simulink model "SkywaveAutopilot"  (R2024b)
settings: Solver=ode45  StartTime=0.0  StopTime=2500  FixedStep=.01  MaxStep=.004  RelTol=1e-5  EnableMultiTasking=on
values from neighbouring files (symbols this model uses):
  ac = [xcg - 0.25 * cbar, 0, 0]    [SkyWaveGeom.m]
  b = 70    [SkyWaveGeom.m]
  cbar = 10    [SkyWaveGeom.m]
  cda2 = 0.33    [SkyWaveGeom.m]
  cdo = 0.05    [SkyWaveGeom.m]
  cg = [xcg 0 0]    [SkyWaveGeom.m]
  cla = 4.44    [SkyWaveGeom.m]
  cladot = 0    [SkyWaveGeom.m]
  clb = -0.074    [SkyWaveGeom.m]
  clda = -0.134    [SkyWaveGeom.m]
  clde = 0.355    [SkyWaveGeom.m]
  cldr = 0.107    [SkyWaveGeom.m]
  clo = 0.41    [SkyWaveGeom.m]
  clp = -0.410    (= -0.41)    [SkyWaveGeom.m]
  clq = 3.8    [SkyWaveGeom.m]
  clr = 0.107    [SkyWaveGeom.m]
  cma = -0.683    [SkyWaveGeom.m]
  cmadot = -4.36    [SkyWaveGeom.m]
  cmde = -0.923    [SkyWaveGeom.m]
  cmq = -9.96    [SkyWaveGeom.m]
  cnb = 0.071    [SkyWaveGeom.m]
  cnda = -0.0035    [SkyWaveGeom.m]
  cndr = -0.072    [SkyWaveGeom.m]
  cnp = -0.0575    [SkyWaveGeom.m]
  cnr = -0.125    [SkyWaveGeom.m]
  cyb = -0.564    [SkyWaveGeom.m]
  cydr = 0.157    [SkyWaveGeom.m]
  eng = [xcg 0 0]    [SkyWaveGeom.m]
  initalt = 5000    [SkyWaveGeom.m]
  initbank = 0    [SkyWaveGeom.m]
  initeast = 0    [SkyWaveGeom.m]
  inithead = 0 * pi / 180    (= 0)    [SkyWaveGeom.m]
  initnorth = 0    [SkyWaveGeom.m]
  initp = 0    [SkyWaveGeom.m]
  initpitch = initw / initu    (= -0.0272251308901)    [SkyWaveGeom.m]
  initq = 0    [SkyWaveGeom.m]
  initr = 0    [SkyWaveGeom.m]
  initu = 238.75    [SkyWaveGeom.m]
  initv = 0    [SkyWaveGeom.m]
  initw = -6.5    [SkyWaveGeom.m]
  jx = 0.25 * mass * (b/2)^2    (= 247282.608696)    [SkyWaveGeom.m]
  jxz = 0    [SkyWaveGeom.m]
  jy = 0.35 * mass * (cbar)^2    (= 28260.8695652)    [SkyWaveGeom.m]
  jz = 0.5 * mass * (b/2)^2    (= 494565.217391)    [SkyWaveGeom.m]
  sw = 700    [SkyWaveGeom.m]
  weight = 26000    [SkyWaveGeom.m]
libraries: slpidlib x7, simulink_extras x5, aerolibfltsims x2, dspswit3 x1, vrlib x1, aerolibanimutils x1
(part 1 of 2)
settings Model: SimulationMode=accelerator  Creator=andersop  LastModifiedBy=gigi
settings SolverCC: InitialStep=.004  AlgebraicLoopSolver=TrustRegion
settings DataIOCC: LimitDataPoints=on  SaveFormat=Array  SignalLoggingSaveFormat=ModelDataLogs  SaveState=on  ReturnWorkspaceOutputs=off  SignalLoggingName=sigsOut
settings OptimizationCC: ExpressionDepthLimit=2147483647  InitFltsAndDblsToZero=on  LifeSpan=inf
settings DebuggingCC: SaveWithParameterizedLinksMsg=none  UnderspecifiedInitializationDetection=Classic  MergeDetectMultiDrivingBlocksExec=none  SignalResolutionControl=TryResolveAllWithWarning  MultiTaskDSMMsg=warning  MultiTaskCondExecSysMsg=none  FcnCallInpInsideContextMsg=warning  UnconnectedInputMsg=warning  UnconnectedOutputMsg=warning  UnconnectedLineMsg=warning  StateNameClashWarn=warning  SFUnexpectedBacktrackingDiag=warning  SFNoUnconditionalDefaultTransitionDiag=warning  SFExecutionAtInitializationDiag=none  ArithmeticOperatorsInVariantConditions=warning
settings HardwareCC: ProdBitPerPointer=32  ProdBitPerSizeT=32  ProdBitPerPtrDiffT=32  ProdLargestAtomicFloat=None  ProdIntDivRoundTo=Undefined  ProdEndianess=Unspecified  ProdWordSize=32  ProdHWDeviceType=32-bit Generic  TargetUnknown=on
settings ModelReferenceCC: PropagateSignalLabelsOutOfModel=off
settings SFSimCC: SimUseLocalCustomCode=off  CustomCodeUndefinedFunction=UseInterfaceOnly
settings RTWCC: RTWUseLocalCustomCode=off  GPUComputeCapability=3.5
settings CodeAppCC: StateflowObjectComments=on
settings GRTTargetCC: TargetFcnLib=ansi_tfl_tmw.mat  TargetLangStandard=C89/C90 (ANSI)  ModelReferenceCompliant=off  CombineOutputUpdateFcns=off  MatFileLogging=off  GRTInterface=on
settings ConfigComp: CovMetricSettings=dw  CovSaveCumulativeToWorkspaceVar=on  CovSaveSingleToWorkspaceVar=on  CovExternalEMLEnable=off

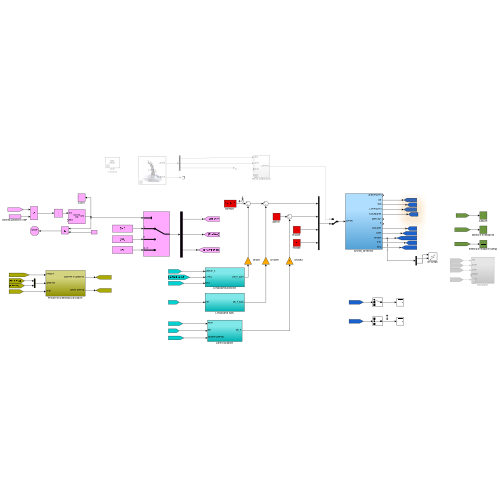
[thumbnail: Simulink's stored preview of the top-level diagram]
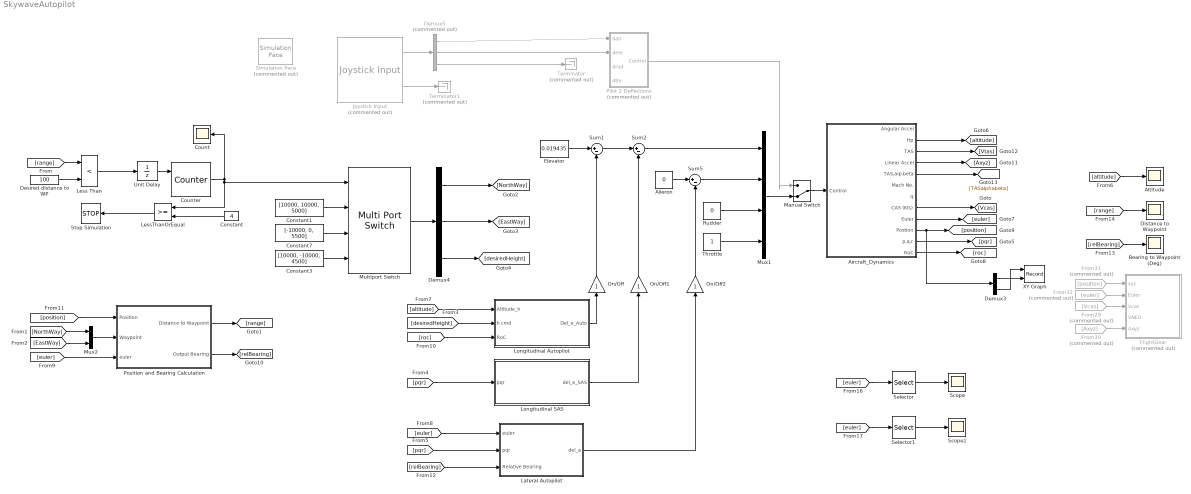
== system SkywaveAutopilot ==
  Aileron : Constant  Value=0
  Aircraft_Dynamics : Subsystem
  Altitude : Scope
  Bearing to Waypoint (Deg) : Scope
  Constant : Constant  Value=4
  Constant1 : Constant  Value=[10000, 10000, 5000]
  Constant3 : Constant  Value=[10000, -10000, 4500]
  Constant7 : Constant  Value=[-10000, 0, 5500]
  Count : Scope
  Counter : dspswit3/Counter  Direction=Up  CountEvent=Rising edge  CounterSize=User defined  MaxCount=255  InitialCount=1  Output=Count  HitValue=32  ResetInput=on  SamplesPerFrame=1  Ts=1  CntDtype=double  HitDtype=Logical
  Demux3 : Demux  Outputs=2
  Demux4 : Demux  Outputs=3
  Demux5 : Demux  Commented=on  Outputs=[1 1 2]
  Desired distance to WP : Constant  Value=100
  Distance to Waypoint : Scope
  Elevator : Constant  Value=0.019435
  FlightGear : Subsystem  Commented=on
  From29 : From  Commented=on  GotoTag=Vcas
  From30 : From  Commented=on  GotoTag=Axyz
  From31 : From  Commented=on  GotoTag=position
  From32 : From  Commented=on  GotoTag=euler
  Joystick Input : vrlib/Joystick Input  Commented=on  joyid=2  adjustports=on  forcefeed=off
  Lateral Autopilot : Subsystem
  Less Than : RelationalOperator  Operator=<  OutDataTypeStr=boolean  RndMeth=Simplest  InputSameDT=off
  LessThanOrEqual : RelationalOperator  OutDataTypeStr=boolean  RndMeth=Simplest  InputSameDT=off
  Longitudinal Autopilot : Subsystem
  Longitudinal SAS : Subsystem
  Manual Switch : ManualSwitch  CurrentSetting=0
  Multiport Switch : MultiPortSwitch  DiagnosticForDefault=None  SaturateOnIntegerOverflow=off  InputSameDT=off
  Mux1 : Mux
  Mux2 : Mux  Inputs=2
  On/Off : Gain
  On/Off1 : Gain
  On/Off2 : Gain
  Pilot 2 Deflections : Subsystem  Commented=on
  Position and Bearing Calculation : Subsystem
  Rudder : Constant  Value=0
  Scope : Scope
  Scope1 : Scope
  Selector : Selector  InputPortWidth=3  IndexOptions=Index vector (dialog)  Indices=[1]  OutputSizes=1
  Selector1 : Selector  InputPortWidth=3  IndexOptions=Index vector (dialog)  Indices=[2]  OutputSizes=1
  Simulation Pace : aerolibanimutils/Simulation Pace  Commented=on  SimulationPace=1  SleepMode=Auto  OutputPaceError=off  SampleTime=1/30
  Stop Simulation : Stop
  Sum1 : Sum  Inputs=|+-
  Sum2 : Sum  Inputs=|+-
  Sum5 : Sum  Inputs=|+-
  Terminator : Terminator  Commented=on
  Terminator1 : Terminator  Commented=on
  Throttle : Constant
  Unit Delay : UnitDelay  InitialCondition=1  SampleTime=-1  HasFrameUpgradeWarning=on
  XY Graph : Record  FileSettingsInternal="{\"entries\":[{\"content\":{\"excelSettings\":{\"content\":{},\"type\":\"Streamout.ExcelSettings\"}},\"type\":\"Streamout.FileSettingStorage\",\"uuid\":\"\"}],\"packageUris\":[\"http:\\/\\/schema.mathworks.com\\/mf0\\/streamout_blocks\\/R2020a\"],\"version\":\"1.0\"}"  Layout=[1 1]  SignalsInternal="{\"entries\":[{\"content\":{\"signals\":[{\"content\":{\"blockPath\":[],\"dimensions\":[1],\"domain\":\"\",\"lineColor\":\"#a2142f\",\"port\":1,\"sid\":[\"\"],\"signalID\":1,\"signalName\":\"Demux3:2\"},\"type\":\"RecordBlkView.Signal\",\"uuid\":\"\"},{\"content\":{\"blockPath\":[],\"dimensions\":[2],\"domain\":\"\",\"hasChildren\":true,\"lineColor\":\"#d95319\",\"lineWidth\":2,\"port\":2,\"sid\":[\"\"],\"signalID\":2,\"signalName\":\"Demux3:1\"},\"type\":\"RecordBlkView.Signal\",\"uuid\":\"\"},{\"content\":{\"blockPath\":[],\"channel\":[1],\"dimensions\":[2],\"domain\":\"\",\"lineColor\":\"#a2142f\",\"lineWidth\":2,\"parentID\":2,\"plots\":[ 1 ],\"port\":2,\"sid\":[\"\"],\"signalID\":3,\"signalName\":\"Demux3:1\"},\"type\":\"RecordBlkView.Signal\",\"uuid\":\"\"},{\"content\":{\"blockPath\":[],\"channel\":[2],\"dimensions\":[2],\"domain\":\"\",\"lineColor\":\"#139fff\",\"lineWidth\":2,\"parentID\":2,\"plots\":[ 1 ],\"port\":2,\"sid\":[\"\"],\"signalID\":4,\"signalName\":\"Demux3:1\"},\"type\":\"RecordBlkView.Signal\",\"uuid\":\"\"}]},\"type\":\"RecordBlkView.InputSignals\",\"uuid\":\"\"}],\"packageUris\":[\"http:\\/\\/schema.mathworks.com\\/mf0\\/streamout_blocks\\/R2020a\"],\"version\":\"1.0\"}"  VisualizationBindings="{\"xyplotplugin\":{\"info\":[{\"series\":[{\"bindingParametersList\":[{\"parameter\":\"X-Axis\",\"signalID\":4,\"signalName\":\"Demux3:1(2)\"},{\"parameter\":\"Y-Axis\",\"signalID\":3,\"signalName\":\"Demux3:1(1)\"}],\"seriesID\":0}],\"subplotID\":1}]}}"  CompatibilityTag=XY
  wires:
  Aircraft_Dynamics/9(Euler) -> [euler]
  Elevator/1 -> Sum1/1
  On/Off/1 -> Sum1/2
  Sum1/1 -> Sum2/1
  On/Off1/1 -> Sum2/2
  Aircraft_Dynamics/10(Postion) -> Demux3/1, [position]
  Position and Bearing Calculation/1(Distance to Waypoint) -> [range]
  Position and Bearing Calculation/2(Output Bearing) -> [relBearing]
  Aileron/1 -> Sum5/1
  Sum5/1 -> Mux1/2
  On/Off2/1 -> Sum5/2
  Lateral Autopilot/1(del_a) -> On/Off2/1
  Counter/1 -> Multiport Switch/1, LessThanOrEqual/1, Count/1
  Less Than/1 -> Unit Delay/1
  Demux3/2 -> XY Graph/1
  Demux3/1 -> XY Graph/2
  Unit Delay/1 -> Counter/1
  Desired distance to WP/1 -> Less Than/2
  Constant/1 -> LessThanOrEqual/2
  LessThanOrEqual/1 -> Stop Simulation/1
  Constant1/1 -> Multiport Switch/2
  Constant7/1 -> Multiport Switch/3
  Constant3/1 -> Multiport Switch/4
  [range] -> Less Than/1
  Multiport Switch/1 -> Demux4/1
  Demux4/1 -> [NorthWay]
  Demux4/2 -> [EastWay]
  Demux4/3 -> [desiredHeight]
  Mux2/1 -> Position and Bearing Calculation/2(Waypoint)
  [NorthWay] -> Mux2/1
  [EastWay] -> Mux2/2
  [desiredHeight] -> Longitudinal Autopilot/2(h cmd)
  Aircraft_Dynamics/11(p,q,r) -> [pqr]
  [pqr] -> Longitudinal SAS/1(pqr)
  [pqr] -> Lateral Autopilot/2(pqr)
  Aircraft_Dynamics/2(Hp) -> [altitude]
  [altitude] -> Altitude/1
  [altitude] -> Longitudinal Autopilot/1(Altitude_h)
  [euler] -> Lateral Autopilot/1(euler)
  [euler] -> Position and Bearing Calculation/3(euler)
  Aircraft_Dynamics/12(RoC) -> [roc]
  [roc] -> Longitudinal Autopilot/3(RoC)
  [position] -> Position and Bearing Calculation/1(Position)
  [relBearing] -> Lateral Autopilot/3(Relative Bearing)
  [relBearing] -> Bearing to Waypoint (Deg)/1
  [range] -> Distance to Waypoint/1
  From32/1 -> FlightGear/2(Euler)
  From31/1 -> FlightGear/1(xyz)
  From29/1 -> FlightGear/3(Vcas)
  From30/1 -> FlightGear/5(Axyz)
  Demux5/2 -> Pilot 2 Deflections/2(dele)
  Joystick Input/2 -> Terminator1/1
  Demux5/3 -> Terminator/1
  Demux5/1 -> Pilot 2 Deflections/1(dail)
  Joystick Input/1 -> Demux5/1
  Mux1/1 -> Manual Switch/2
  Pilot 2 Deflections/1(Control) -> Manual Switch/1
  Manual Switch/1 -> Aircraft_Dynamics/1(Control)
  Aircraft_Dynamics/8(CAS (Kts)) -> [Vcas]
  Aircraft_Dynamics/4(Linear Accel) -> [Axyz]
  Aircraft_Dynamics/3(TAS) -> [Vtas]
  [euler] -> Selector/1
  Selector/1 -> Scope/1
  [euler] -> Selector1/1
  Selector1/1 -> Scope1/1
  Rudder/1 -> Mux1/3
  Sum2/1 -> Mux1/1
  Throttle/1 -> Mux1/4
  Longitudinal Autopilot/1(Del_e_Auto) -> On/Off/1
  Longitudinal SAS/1(del_e_SAS) -> On/Off1/1
  Aircraft_Dynamics/5(TAS,alp,beta) -> [TASalphabeta]

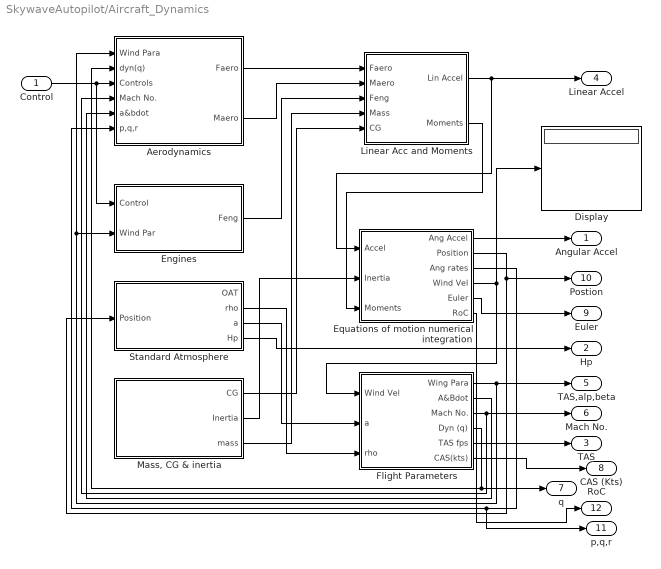
== system SkywaveAutopilot/Aircraft_Dynamics ==
  Control : Inport
  Aerodynamics : Subsystem
  Display : Display
  Engines : Subsystem
  "Equations of motion numerical integration " : Subsystem
  Flight Parameters : Subsystem
  Linear Acc and Moments : Subsystem
  "Mass, CG & inertia" : Subsystem
  Standard Atmosphere : Subsystem
  Angular Accel : Outport
  Hp : Outport  Port=2
  TAS : Outport  Port=3
  Linear Accel : Outport  Port=4
  TAS,alp,beta : Outport  Port=5
  Mach No. : Outport  Port=6
  q : Outport  Port=7
  CAS (Kts) : Outport  Port=8
  Euler : Outport  Port=9
  Postion : Outport  Port=10
  p,q,r : Outport  Port=11
  RoC : Outport  Port=12
  wires:
  Aerodynamics/1(Faero) -> Linear Acc and Moments/1(Faero)
  Aerodynamics/2(Maero) -> Linear Acc and Moments/2(Maero)
  Control/1 -> Aerodynamics/3(Controls), Engines/1(Control)
  Engines/1(Feng) -> Linear Acc and Moments/3(Feng)
  "Mass, CG & inertia"/1(CG) -> Linear Acc and Moments/5(CG)
  "Mass, CG & inertia"/2(Inertia) -> "Equations of motion numerical integration "/2(Inertia)
  Linear Acc and Moments/1(Lin Accel) -> "Equations of motion numerical integration "/1(Accel), Linear Accel/1
  Linear Acc and Moments/2(Moments) -> "Equations of motion numerical integration "/3(Moments)
  "Equations of motion numerical integration "/3(Ang rates) -> Aerodynamics/6(p,q,r), p,q,r/1
  "Equations of motion numerical integration "/4(Wind Vel) -> Display/1, Flight Parameters/1(Wind Vel)
  Flight Parameters/1(Wing Para) -> TAS,alp,beta/1, Aerodynamics/1(Wind Para), Engines/2(Wind Par)
  Flight Parameters/4(Dyn (q)) -> Aerodynamics/2(dyn(q)), q/1
  Flight Parameters/3(Mach No.) -> Mach No./1, Aerodynamics/4(Mach No.)
  Flight Parameters/2(A&Bdot) -> Aerodynamics/5(a&bdot)
  "Equations of motion numerical integration "/2(Position) -> Postion/1, Standard Atmosphere/1(Position)
  "Equations of motion numerical integration "/1(Ang Accel) -> Angular Accel/1
  Standard Atmosphere/4(Hp) -> Hp/1
  Flight Parameters/5(TAS fps) -> TAS/1
  Flight Parameters/6(CAS(kts)) -> CAS (Kts)/1
  "Equations of motion numerical integration "/5(Euler) -> Euler/1
  Standard Atmosphere/3(a) -> Flight Parameters/2(a)
  Standard Atmosphere/2(rho) -> Flight Parameters/3(rho)
  "Mass, CG & inertia"/3(mass) -> Linear Acc and Moments/4(Mass)
  "Equations of motion numerical integration "/6(RoC) -> RoC/1

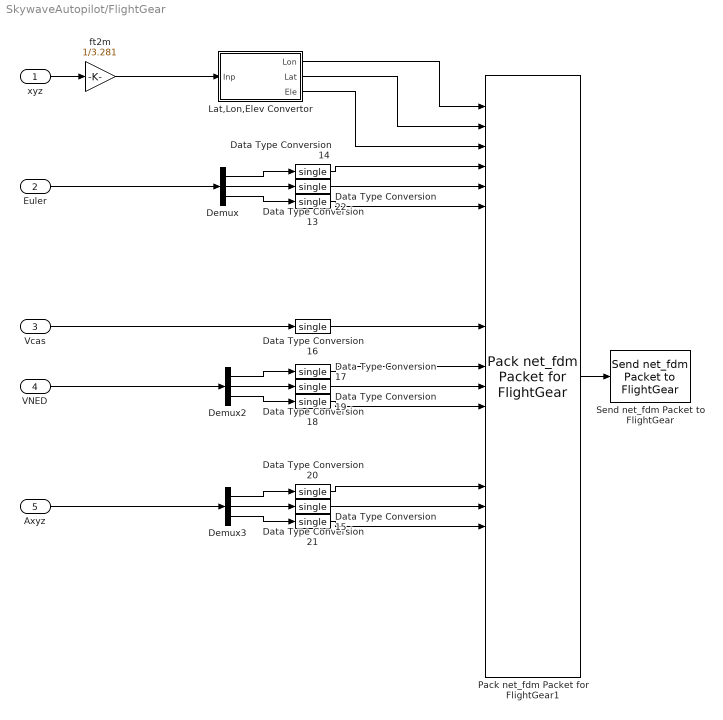
== system SkywaveAutopilot/FlightGear ==
  xyz : Inport
  Euler : Inport  Port=2
  Vcas : Inport  Port=3
  VNED : Inport  Port=4
  Axyz : Inport  Port=5
  Data Type Conversion{13..22} (10 alike) : DataTypeConversion  OutDataTypeStr=single  SaturateOnIntegerOverflow=off  RndMeth=Floor
  Demux : Demux  Outputs=3
  Demux2 : Demux  Outputs=3
  Demux3 : Demux  Outputs=3
  Lat,Lon,Elev Convertor : Subsystem  mask{lat_ref=37.7212*pi/180, long_ref=-122.2236*pi/180, h_ref=0}
      mask prompts: lat_ref "Initial latitude"; long_ref "Initial longitude"; h_ref "Intial altitude"
      mask DialogControl DescTextVar Prompt: Convert x,y,z coordinates (in m) to latitude, longitude and altitude.
  Pack net_fdm Packet for FlightGear1 : aerolibfltsims/Pack net_fdm Packet for FlightGear  FlightGearVersion=v2.4  ShowPositionAttitudeInputs=on  ShowVelocityAccelerationInputs=on  ShowControlSurfacePositionInputs=off  ShowEngineFuelInputs=off  ShowLandingGearInputs=off  ShowEnvironmentInputs=on  SampleTime=-1  packetVersion=24
  Send net_fdm Packet to FlightGear : aerolibfltsims/Send net_fdm Packet to FlightGear  DestinationIpAddress=127.0.0.1  DestinationPort=5502  LocalIpPort=-1  varLen=off  SampleTime=-1
  ft2m : Gain  Gain=1/3.281
  wires:
  xyz/1 -> ft2m/1
  Demux/1 -> Data Type Conversion14/1
  Demux2/2 -> Data Type Conversion18/1
  Demux2/3 -> Data Type Conversion19/1
  Lat,Lon,Elev Convertor/2(Lat) -> Pack net_fdm Packet for FlightGear1/2
  Vcas/1 -> Data Type Conversion16/1
  Data Type Conversion18/1 -> Pack net_fdm Packet for FlightGear1/15
  Demux3/1 -> Data Type Conversion20/1
  Demux/3 -> Data Type Conversion22/1
  Pack net_fdm Packet for FlightGear1/1 -> Send net_fdm Packet to FlightGear/1
  Demux3/2 -> Data Type Conversion21/1
  Data Type Conversion14/1 -> Pack net_fdm Packet for FlightGear1/4
  Data Type Conversion16/1 -> Pack net_fdm Packet for FlightGear1/12
  Data Type Conversion19/1 -> Pack net_fdm Packet for FlightGear1/16
  Demux2/1 -> Data Type Conversion17/1
  Data Type Conversion17/1 -> Pack net_fdm Packet for FlightGear1/14
  Data Type Conversion13/1 -> Pack net_fdm Packet for FlightGear1/5
  Demux3/3 -> Data Type Conversion15/1
  Lat,Lon,Elev Convertor/1(Lon) -> Pack net_fdm Packet for FlightGear1/1
  Demux/2 -> Data Type Conversion13/1
  Data Type Conversion22/1 -> Pack net_fdm Packet for FlightGear1/6
  Data Type Conversion15/1 -> Pack net_fdm Packet for FlightGear1/22
  Data Type Conversion21/1 -> Pack net_fdm Packet for FlightGear1/21
  Data Type Conversion20/1 -> Pack net_fdm Packet for FlightGear1/20
  Euler/1 -> Demux/1
  VNED/1 -> Demux2/1
  Axyz/1 -> Demux3/1
  ft2m/1 -> Lat,Lon,Elev Convertor/1(Inp)
  Lat,Lon,Elev Convertor/3(Ele) -> Pack net_fdm Packet for FlightGear1/3

== system SkywaveAutopilot/Lateral Autopilot ==
  euler : Inport
  pqr : Inport  Port=2
  Relative Bearing : Inport  Port=3
  Degrees to Radians2 : simulink_extras/Transformations/Degrees to Radians
  PID Controller : slpidlib/PID Controller  Controller=PID  Form=Parallel  TimeDomain=Continuous-time  UseExternalTs=off  SampleTime=-1  IntegratorMethod=Forward Euler  FilterMethod=Forward Euler  ControllerParametersSource=internal  P=-0.02395958051733  I=-0.000320661654489458  UseKiTs=off  D=-0.419646250654046  UseExternalDerivativeSource=off  N=0.858384035083812  UseFilter=on  TunerSelectOption=Transfer Function Based (PID Tuner App)  InitialConditionSource=internal  InitialConditionForIntegrator=0  InitialConditionForFilter=0  DifferentiatorICPrevScaledInput=0  ExternalReset=none  TrackingMode=off  Kt=1  LimitOutput=off  SatLimitsSource=internal  UpperSaturationLimit=inf  LowerSaturationLimit=-inf  LinearizeAsGain=on  AntiWindupMode=none  Kb=1  LimitIntegrator=off  UpperIntegratorSaturationLimit=inf  LowerIntegratorSaturationLimit=-inf  POutMin=[]  POutMax=[]  IOutMin=[]  IOutMax=[]  DOutMin=[]  DOutMax=[]  NOutMin=[]  NOutMax=[]  SumOutMin=[]  SumOutMax=[]  SaturationOutMin=[]  SaturationOutMax=[]  PParamMin=[]  PParamMax=[]  IParamMin=[]  IParamMax=[]  DParamMin=[]  DParamMax=[]  NParamMin=[]  NParamMax=[]  KbParamMin=[]  KbParamMax=[]  KtParamMin=[]  KtParamMax=[]  KbOutMin=[]  KbOutMax=[]  KtOutMin=[]  KtOutMax=[]  IntegratorOutMin=[]  IntegratorOutMax=[]  FilterOutMin=[]  FilterOutMax=[]  SumI1OutMin=[]  SumI1OutMax=[]  SumI2OutMin=[]  SumI2OutMax=[]  SumI3OutMin=[]  SumI3OutMax=[]  SumI4OutMin=[]  SumI4OutMax=[]  SumDOutMin=[]  SumDOutMax=[]  DifferentiatorOutMin=[]  DifferentiatorOutMax=[]  FilterDiffOutCoefMin=[]  FilterDiffOutCoefMax=[]  ReciprocalOutMin=[]  ReciprocalOutMax=[]  SumDenOutMin=[]  SumDenOutMax=[]  SumNumOutMin=[]  SumNumOutMax=[]  DivideOutMin=[]  DivideOutMax=[]  UdiffTsProdOutMin=[]  UdiffTsProdOutMax=[]  NTsProdOutMin=[]  NTsProdOutMax=[]  UintegralTsProdOutMin=[]  UintegralTsProdOutMax=[]  UngainTsProdOutMin=[]  UngainTsProdOutMax=[]  ClampingZeroOutDataTypeStr=Inherit: Inherit via back propagation  ClampingZeroOutMin=[]  ClampingZeroOutMax=[]  FilterDenConstantOutDataTypeStr=Inherit: Inherit via back propagation  FilterDenConstantOutMin=[]  FilterDenConstantOutMax=[]  PCopyOutDataTypeStr=Inherit: Inherit via back propagation  PCopyOutMin=[]  PCopyOutMax=[]  NCopyOutDataTypeStr=Inherit: Inherit via back propagation  NCopyOutMin=[]  NCopyOutMax=[]  IntegratorContinuousStateAttributes=''  IntegratorStateMustResolveToSignalObject=off  IntegratorRTWStateStorageClass=Auto  FilterContinuousStateAttributes=''  FilterStateMustResolveToSignalObject=off  FilterRTWStateStorageClass=Auto  ParallelPVariant=InternalParameters  IdealPVariant=Disabled  IVariant=InternalParameters  DVariant=InternalParameters  IntegratorVariant=Continuous  SatVariant=Disabled  AWVariant=Passthrough  PCopyVariant=Disabled  TRVariant=Disabled  FdbkBlocksVariant=Forward  IdealPFdbkVariant=Disabled  SatFdbkVariant=Disabled  DerivativeFilterVariant=ContFilter  NVariant=InternalParameters  NCopyVariant=Disabled  FilterICVariant=InternalICsFilter  IntegratorICVariant=InternalICs  ExternalResetVariant=Disabled  TRSumVariant=Passthrough  SumFdbkVariant=Disabled  SumVariant=Sum_PID  TsampFilterVariant=InternalTs  TsampNgainVariant=Passthrough  TsampIntegralVariant=Disabled_SignalSpec  ExternalSaturationOutDataTypeStr=Inherit: Same as second input  DerivativeSourceVariant=ErrorSignal  PreIntVariant=InternalPreInt
  P_CMD1 : Lookup_n-D  NumberOfTableDimensions=1  BreakpointsForDimension1=[-180 -10 0 10 180]  Table=[-10 -10 0 10 10]  InternalRulePriority=Speed  RndMeth=Simplest
  Phi_CMD2 : Lookup_n-D  NumberOfTableDimensions=1  BreakpointsForDimension1=[-180 -10 0 10 180]  Table=[-17 -17 0 17 17]  InternalRulePriority=Speed  RndMeth=Simplest
  Radians to Degrees1 : simulink_extras/Transformations/Radians to Degrees
  Selector : Selector  InputPortWidth=3  IndexOptions=Index vector (dialog)  Indices=1  OutputSizes=1
  Selector1 : Selector  InputPortWidth=3  IndexOptions=Index vector (dialog)  Indices=1  OutputSizes=1
  Sum3 : Sum  Inputs=|+-
  Sum4 : Sum  Inputs=|+-
  del_a : Outport
  wires:
  Sum4/1 -> PID Controller/1
  euler/1 -> Selector1/1
  Relative Bearing/1 -> Phi_CMD2/1
  pqr/1 -> Selector/1
  PID Controller/1 -> del_a/1
  P_CMD1/1 -> Sum4/2
  Selector/1 -> Sum4/1
  Selector1/1 -> Sum3/2
  Phi_CMD2/1 -> Degrees to Radians2/1
  Degrees to Radians2/1 -> Sum3/1
  Sum3/1 -> Radians to Degrees1/1
  Radians to Degrees1/1 -> P_CMD1/1

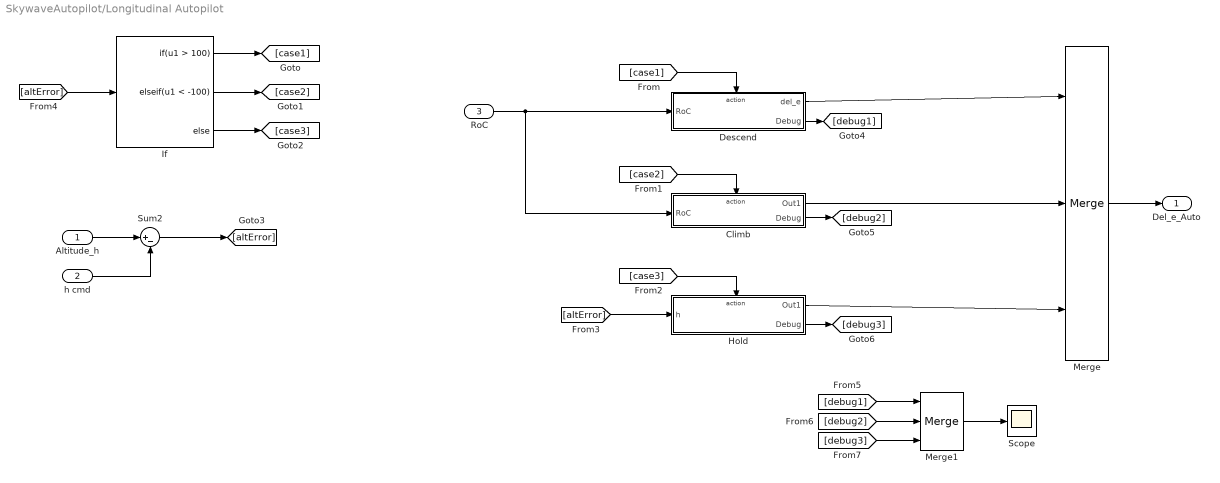
== system SkywaveAutopilot/Longitudinal Autopilot ==
  Altitude_h : Inport
  h cmd : Inport  Port=2
  RoC : Inport  Port=3
  Climb : Subsystem  TreatAsAtomicUnit=on
  Descend : Subsystem  TreatAsAtomicUnit=on
  Hold : Subsystem  TreatAsAtomicUnit=on
  If : If  IfExpression=u1 > 100  ElseIfExpressions=u1 < -100
  Merge : Merge  Inputs=3
  Merge1 : Merge  Inputs=3
  Scope : Scope
  Sum2 : Sum  Inputs=|+-
  Del_e_Auto : Outport
  wires:
  Altitude_h/1 -> Sum2/1
  RoC/1 -> Climb/1(RoC), Descend/1(RoC)
  Descend/1(del_e) -> Merge/1
  Merge/1 -> Del_e_Auto/1
  Hold/1(Out1) -> Merge/3
  Climb/1(Out1) -> Merge/2
  Merge1/1 -> Scope/1
  h cmd/1 -> Sum2/2
  If/1 -> [case1]
  If/2 -> [case2]
  If/3 -> [case3]
  [case3] -> Hold/Action
  [case2] -> Climb/Action
  [case1] -> Descend/Action
  Sum2/1 -> [altError]
  [altError] -> Hold/1(h)
  [altError] -> If/1
  Descend/2(Debug) -> [debug1]
  Climb/2(Debug) -> [debug2]
  Hold/2(Debug) -> [debug3]
  [debug3] -> Merge1/3
  [debug1] -> Merge1/1
  [debug2] -> Merge1/2

== system SkywaveAutopilot/Longitudinal SAS ==
  pqr : Inport
  Desired q : Constant  Value=0
  SAS Gain : Gain  Gain=-3
  Selector : Selector  InputPortWidth=3  IndexOptions=Index vector (dialog)  Indices=2  OutputSizes=1
  Sum1 : Sum  Inputs=|+-
  del_e_SAS : Outport
  wires:
  Sum1/1 -> SAS Gain/1
  Desired q/1 -> Sum1/2
  SAS Gain/1 -> del_e_SAS/1
  pqr/1 -> Selector/1
  Selector/1 -> Sum1/1

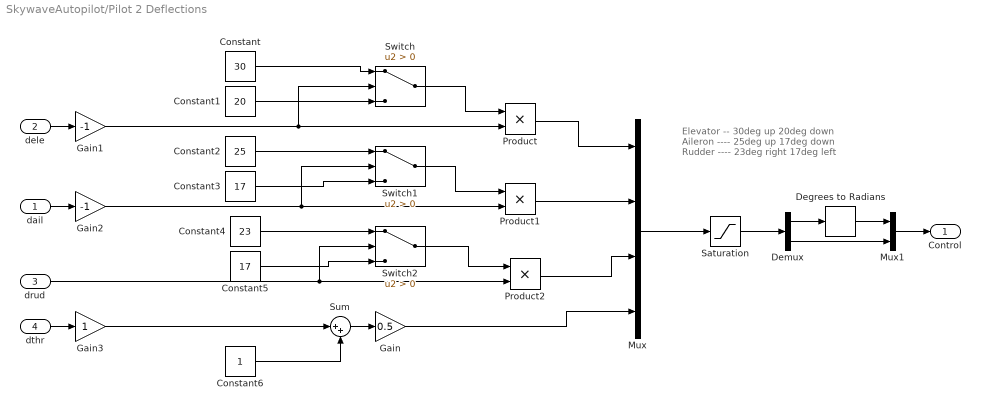
== system SkywaveAutopilot/Pilot 2 Deflections ==
  note: Elevator -- 30deg up     20deg down
      | Aileron ---- 25deg up     17deg down
      | Rudder ---- 23deg right  17deg left
  dail : Inport
  dele : Inport  Port=2
  drud : Inport  Port=3
  dthr : Inport  Port=4
  Constant : Constant  Value=30
  Constant1 : Constant  Value=20
  Constant2 : Constant  Value=25
  Constant3 : Constant  Value=17
  Constant4 : Constant  Value=23
  Constant5 : Constant  Value=17
  Constant6 : Constant
  Degrees to Radians : simulink_extras/Transformations/Degrees to Radians
  Demux : Demux  Outputs=[3 1]
  Gain : Gain  Gain=0.5
  Gain1 : Gain  Gain=-1
  Gain2 : Gain  Gain=-1
  Gain3 : Gain
  Mux : Mux
  Mux1 : Mux  Inputs=2
  Product : Product
  Product1 : Product
  Product2 : Product
  Saturation : Saturate  UpperLimit=[30 25 23 1]  LowerLimit=[-20 -17 -17 0]
  Sum : Sum  Inputs=|++
  Switch : Switch  Criteria=u2 > Threshold  SaturateOnIntegerOverflow=off  InputSameDT=off
  Switch1 : Switch  Criteria=u2 > Threshold  SaturateOnIntegerOverflow=off  InputSameDT=off
  Switch2 : Switch  Criteria=u2 > Threshold  SaturateOnIntegerOverflow=off  InputSameDT=off
  Control : Outport
  wires:
  Mux/1 -> Saturation/1
  dele/1 -> Gain1/1
  Gain1/1 -> Switch/2, Product/2
  Switch/1 -> Product/1
  Constant1/1 -> Switch/3
  Constant/1 -> Switch/1
  Product/1 -> Mux/1
  Constant2/1 -> Switch1/1
  Constant3/1 -> Switch1/3
  Switch1/1 -> Product1/1
  Gain2/1 -> Product1/2, Switch1/2
  dail/1 -> Gain2/1
  Product1/1 -> Mux/2
  Gain3/1 -> Sum/1
  dthr/1 -> Gain3/1
  Sum/1 -> Gain/1
  Constant6/1 -> Sum/2
  Gain/1 -> Mux/4
  Mux1/1 -> Control/1
  Saturation/1 -> Demux/1
  Demux/1 -> Degrees to Radians/1
  Degrees to Radians/1 -> Mux1/1
  Demux/2 -> Mux1/2
  drud/1 -> Switch2/2, Product2/2
  Product2/1 -> Mux/3
  Switch2/1 -> Product2/1
  Constant5/1 -> Switch2/3
  Constant4/1 -> Switch2/1

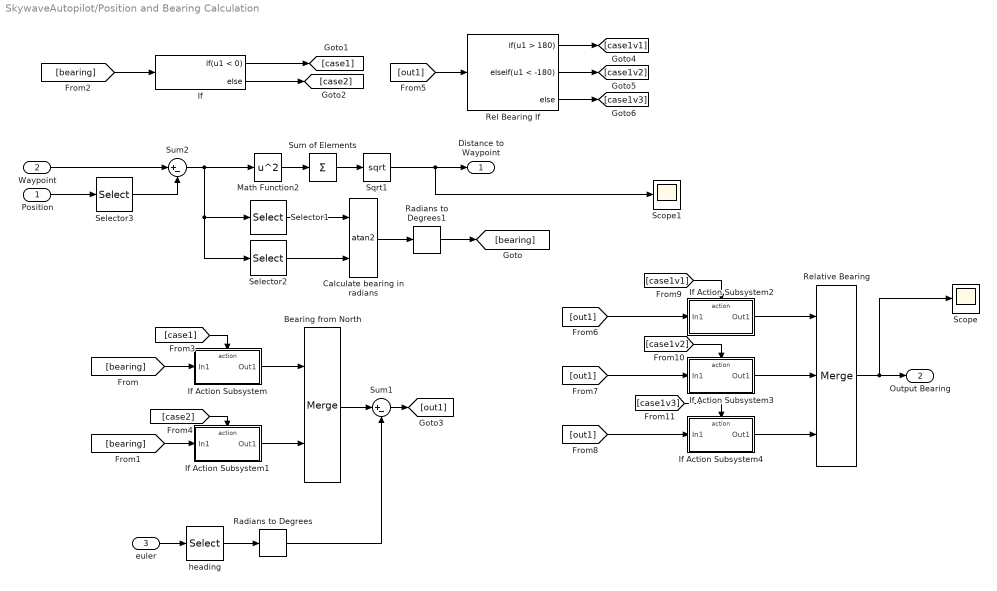
== system SkywaveAutopilot/Position and Bearing Calculation ==
  Position : Inport
  Waypoint : Inport  Port=2
  euler : Inport  Port=3
  Bearing from North : Merge
  Calculate bearing in radians : Trigonometry  Operator=atan2
  If : If  IfExpression=u1 < 0
  If Action Subsystem : Subsystem  TreatAsAtomicUnit=on
  If Action Subsystem1 : Subsystem  TreatAsAtomicUnit=on
  If Action Subsystem2 : Subsystem  TreatAsAtomicUnit=on
  If Action Subsystem3 : Subsystem  TreatAsAtomicUnit=on
  If Action Subsystem4 : Subsystem  TreatAsAtomicUnit=on
  Math Function2 : Math  Operator=square
  Radians to Degrees : simulink_extras/Transformations/Radians to Degrees
  Radians to Degrees1 : simulink_extras/Transformations/Radians to Degrees
  Rel Bearing If : If  IfExpression=u1 > 180  ElseIfExpressions=u1 < -180
  Relative Bearing : Merge  Inputs=3
  Scope : Scope
  Scope1 : Scope
  Selector1 : Selector  InputPortWidth=2  IndexOptions=Index vector (dialog)  Indices=2  OutputSizes=1
  Selector2 : Selector  InputPortWidth=2  IndexOptions=Index vector (dialog)  Indices=1  OutputSizes=1
  Selector3 : Selector  InputPortWidth=3  IndexOptions=Index vector (dialog)  Indices=[1 2]  OutputSizes=1
  Sqrt1 : Sqrt
  Sum of Elements : Sum  Inputs=+
  Sum1 : Sum  Inputs=|+-
  Sum2 : Sum  Inputs=|+-
  heading : Selector  InputPortWidth=3  IndexOptions=Index vector (dialog)  Indices=[3]  OutputSizes=1
  Distance to Waypoint : Outport
  Output Bearing : Outport  Port=2
  wires:
  Waypoint/1 -> Sum2/1
  Position/1 -> Selector3/1
  Calculate bearing in radians/1 -> Radians to Degrees1/1
  Bearing from North/1 -> Sum1/1
  If Action Subsystem/1(Out1) -> Bearing from North/1
  If Action Subsystem1/1(Out1) -> Bearing from North/2
  If Action Subsystem2/1(Out1) -> Relative Bearing/1
  If Action Subsystem3/1(Out1) -> Relative Bearing/2
  If Action Subsystem4/1(Out1) -> Relative Bearing/3
  Relative Bearing/1 -> Scope/1, Output Bearing/1
  euler/1 -> heading/1
  heading/1 -> Radians to Degrees/1
  Radians to Degrees/1 -> Sum1/2
  Sum of Elements/1 -> Sqrt1/1
  Sqrt1/1 -> Scope1/1, Distance to Waypoint/1
  Math Function2/1 -> Sum of Elements/1
  Sum2/1 -> Selector2/1, Selector1/1, Math Function2/1
  Selector1/1 -> Calculate bearing in radians/1
  Selector2/1 -> Calculate bearing in radians/2
  Selector3/1 -> Sum2/2
  Radians to Degrees1/1 -> [bearing]
  [bearing] -> If Action Subsystem/1(In1)
  [bearing] -> If Action Subsystem1/1(In1)
  [bearing] -> If/1
  If/1 -> [case1]
  If/2 -> [case2]
  [case1] -> If Action Subsystem/Action
  [case2] -> If Action Subsystem1/Action
  Sum1/1 -> [out1]
  [out1] -> Rel Bearing If/1
  [out1] -> If Action Subsystem2/1(In1)
  [out1] -> If Action Subsystem3/1(In1)
  [out1] -> If Action Subsystem4/1(In1)
  Rel Bearing If/1 -> [case1v1]
  Rel Bearing If/2 -> [case1v2]
  Rel Bearing If/3 -> [case1v3]
  [case1v1] -> If Action Subsystem2/Action
  [case1v2] -> If Action Subsystem3/Action
  [case1v3] -> If Action Subsystem4/Action

== system SkywaveAutopilot/Aircraft_Dynamics/Aerodynamics ==
  note: Notes: alpha is measured from
  Wind Para : Inport
  dyn(q) : Inport  Port=2
  Controls : Inport  Port=3
  Mach No. : Inport  Port=4
  a&bdot : Inport  Port=5
  p,q,r : Inport  Port=6
  Aero Forces and Moments : Subsystem
  CD : Subsystem
  CL : Subsystem
  CM : Subsystem
  CN : Subsystem
  CY : Subsystem
  Croll : Subsystem
  Faero : Outport
  Maero : Outport  Port=2
  wires:
  Wind Para/1 -> CL/1(Wind Parameters), CY/1(Wind Parameters), Aero Forces and Moments/5(Wind Para), CN/1(Wind Parameters), Croll/1(Wind Parameters), CM/1(Wind Parameters), CD/1(Wind Parameters)
  CL/1(CL) -> Aero Forces and Moments/4(CL)
  Mach No./1 -> CM/3(Mach No.), CN/3(Mach No.), Croll/3(Mach No.), CY/3(Mach No.), CL/3(Mach No.), CD/3(Mach No.)
  a&bdot/1 -> CL/4(a&bdot), CM/4(a&bdot)
  p,q,r/1 -> CM/5(P,q,r), CN/4(P,q,r), Croll/4(P,q,r), CY/4(P,q,r), CL/5(P,q,r)
  Controls/1 -> CM/2(Controls), CD/2(Controls), CN/2(Controls), Croll/2(Controls), CY/2(Controls), CL/2(Controls)
  CD/1(CD) -> Aero Forces and Moments/2(CD)
  CN/1(CN) -> Aero Forces and Moments/8(CN)
  Croll/1(Croll) -> Aero Forces and Moments/6(Croll)
  CY/1(CY) -> Aero Forces and Moments/3(CY)
  CM/1(CM) -> Aero Forces and Moments/7(CM)
  dyn(q)/1 -> Aero Forces and Moments/1(dyn(q))
  Aero Forces and Moments/1(Faero) -> Faero/1
  Aero Forces and Moments/2(Maero) -> Maero/1

== system SkywaveAutopilot/Aircraft_Dynamics/Engines ==
  Control : Inport
  Wind Par : Inport  Port=2
  Demux : Demux
  Demux1 : Demux  Outputs=3
  Display : Display
  Max Power : Constant  Value=200*550
  Product : Product  RndMeth=Zero
  Product1 : Product  Inputs=*/  RndMeth=Zero
  Terminator{,1..4} (5 alike) : Terminator
  Feng : Outport
  wires:
  Max Power/1 -> Product/2
  Control/1 -> Demux/1
  Demux/4 -> Product/1
  Demux/1 -> Terminator/1
  Demux/2 -> Terminator1/1
  Demux/3 -> Terminator2/1
  Product/1 -> Product1/1
  Product1/1 -> Feng/1, Display/1
  Wind Par/1 -> Demux1/1
  Demux1/1 -> Product1/2
  Demux1/2 -> Terminator4/1
  Demux1/3 -> Terminator3/1

== system SkywaveAutopilot/Aircraft_Dynamics/Equations of motion numerical integration  ==
  Accel : Inport
  Inertia : Inport  Port=2
  Moments : Inport  Port=3
  Flat Earth Navigation : Subsystem
  Force Equations : Subsystem
  Gravity Model : Subsystem
  Inert-body : Subsystem
  Kinematic Equiations : Subsystem
  Moment Equations : Subsystem
  Ang Accel : Outport
  Position : Outport  Port=2
  Ang rates : Outport  Port=3
  Wind Vel : Outport  Port=4
  Euler : Outport  Port=5
  RoC : Outport  Port=6
  wires:
  Moment Equations/1(Ang Rates) -> Ang rates/1, Kinematic Equiations/1(Rates), Force Equations/3(Rates)
  Kinematic Equiations/1(Euler angles) -> Flat Earth Navigation/1(Euler Angles), Inert-body/1(Euler), Euler/1
  Force Equations/1(Lin Vel) -> Wind Vel/1, Flat Earth Navigation/2(Velocity)
  Accel/1 -> Force Equations/1(Accel)
  Inertia/1 -> Moment Equations/1(Inertia)
  Gravity Model/1(Gravity) -> Force Equations/2(Gravity)
  Moments/1 -> Moment Equations/2(Moments)
  Moment Equations/2(Ang Accel) -> Ang Accel/1
  Flat Earth Navigation/1(Position) -> Position/1
  Inert-body/1(NEDtoBC) -> Force Equations/4(NEDtoABC)
  Flat Earth Navigation/2(RoC) -> RoC/1

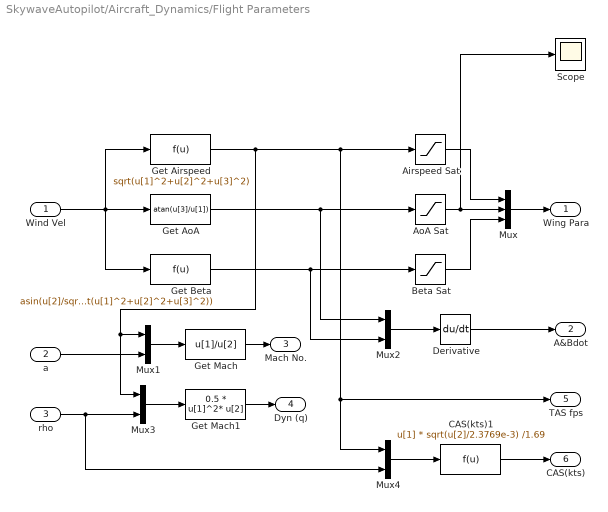
== system SkywaveAutopilot/Aircraft_Dynamics/Flight Parameters ==
  Wind Vel : Inport
  a : Inport  Port=2
  rho : Inport  Port=3
  Airspeed Sat : Saturate  UpperLimit=1100  LowerLimit=0  ZeroCross=off
  AoA Sat : Saturate  UpperLimit=0.3  LowerLimit=-0.2  ZeroCross=off
  Beta Sat : Saturate  UpperLimit=0.4  LowerLimit=-0.4  ZeroCross=off
  CAS(kts)1 : Fcn  Expr=u[1] * sqrt(u[2]/2.3769e-3) /1.69
  Derivative : Derivative
  Get Airspeed : Fcn  Expr=sqrt(u[1]^2+u[2]^2+u[3]^2)
  Get AoA : Fcn  Expr=atan(u[3]/u[1])
  Get Beta : Fcn  Expr=asin(u[2]/sqrt(u[1]^2+u[2]^2+u[3]^2))
  Get Mach : Fcn  Expr=u[1]/u[2]
  Get Mach1 : Fcn  Expr=0.5 * u[1]^2* u[2]
  Mux : Mux  Inputs=3
  Mux{1..4} (4 alike) : Mux  Inputs=2
  Scope : Scope
  Wing Para : Outport
  A&Bdot : Outport  Port=2
  Mach No. : Outport  Port=3
  Dyn (q) : Outport  Port=4
  TAS fps : Outport  Port=5
  CAS(kts) : Outport  Port=6
  wires:
  Wind Vel/1 -> Get AoA/1, Get Airspeed/1, Get Beta/1
  Get Airspeed/1 -> Mux1/1, Mux3/1, Airspeed Sat/1, TAS fps/1, Mux4/1
  Get AoA/1 -> AoA Sat/1, Mux2/1
  Get Beta/1 -> Beta Sat/1, Mux2/2
  AoA Sat/1 -> Mux/2, Scope/1
  Airspeed Sat/1 -> Mux/1
  Beta Sat/1 -> Mux/3
  Mux/1 -> Wing Para/1
  Mux1/1 -> Get Mach/1
  a/1 -> Mux1/2
  Mux2/1 -> Derivative/1
  Derivative/1 -> A&Bdot/1
  Get Mach/1 -> Mach No./1
  rho/1 -> Mux3/2, Mux4/2
  Mux3/1 -> Get Mach1/1
  Get Mach1/1 -> Dyn (q)/1
  Mux4/1 -> CAS(kts)1/1
  CAS(kts)1/1 -> CAS(kts)/1

== system SkywaveAutopilot/Aircraft_Dynamics/Linear Acc and Moments ==
  Faero : Inport
  Maero : Inport  Port=2
  Feng : Inport  Port=3
  Mass : Inport  Port=4
  CG : Inport  Port=5
  Aero Center : Constant  Value=ac
  Cross Prod Moment due Leng : Subsystem
  Cross Prod Moment due to Aero : Subsystem
  DngPOS : Constant  Value=eng
  F/m : Product  Inputs=*/  SaturateOnIntegerOverflow=on  OutDataTypeStr=Inherit: Same as first input
  Mux : Mux  Inputs=3
  Scope1 : Scope
  Sum1 : Sum  SaturateOnIntegerOverflow=on
  Sum2 : Sum  Inputs=|+-  SaturateOnIntegerOverflow=on
  Sum4 : Sum  Inputs=+++  SaturateOnIntegerOverflow=on
  Sum5 : Sum  Inputs=|+-  SaturateOnIntegerOverflow=on
  Thrust Y&Z : Constant  Value=0
  Lin Accel : Outport
  Moments : Outport  Port=2
  wires:
  Feng/1 -> Cross Prod Moment due Leng/2(Vec 2), Mux/1
  Thrust Y&Z/1 -> Mux/2, Mux/3
  Faero/1 -> Sum1/1, Cross Prod Moment due to Aero/2(Vec 2)
  Mux/1 -> Sum1/2
  Sum1/1 -> F/m/1
  Mass/1 -> F/m/2
  F/m/1 -> Lin Accel/1
  CG/1 -> Sum2/2, Sum5/2
  Aero Center/1 -> Sum5/1
  Sum5/1 -> Cross Prod Moment due to Aero/1(Vec 1)
  Maero/1 -> Sum4/2
  Sum4/1 -> Moments/1
  Cross Prod Moment due to Aero/1(X Prod) -> Sum4/1
  Sum2/1 -> Cross Prod Moment due Leng/1(Vec 1)
  Cross Prod Moment due Leng/1(X Prod) -> Sum4/3, Scope1/1
  DngPOS/1 -> Sum2/1

== system SkywaveAutopilot/Aircraft_Dynamics/Mass, CG & inertia ==
  Mux1 : Mux
  cg : Constant  Value=cg
  jx : Constant  Value=jx
  jxz : Constant  Value=jxz
  jy : Constant  Value=jy
  jz : Constant  Value=jz
  mass2 : Constant  Value=weight/32.2
  CG : Outport
  Inertia : Outport  Port=2
  mass : Outport  Port=3
  wires:
  cg/1 -> CG/1
  jy/1 -> Mux1/2
  jx/1 -> Mux1/1
  jz/1 -> Mux1/3
  jxz/1 -> Mux1/4
  Mux1/1 -> Inertia/1
  mass2/1 -> mass/1

== system SkywaveAutopilot/Aircraft_Dynamics/Standard Atmosphere ==
  Position : Inport
  Demux : Demux  Outputs=3
      settings: DisplayOption=none
  Density : Fcn  Expr=2.3769e-3*(1 - 0.703e-5 * u[1])^4.14
  OATemp : Lookup  InputValues=[0 35000 60000]  Table=[519 390 390]
  Speed of Sound : Fcn  Expr=sqrt(1.4*1716.3*u[1])
  Terminator : Terminator
  Terminator1 : Terminator
  OAT : Outport
  rho : Outport  Port=2
  a : Outport  Port=3
  Hp : Outport  Port=4
  wires:
  OATemp/1 -> OAT/1, Speed of Sound/1
  Density/1 -> rho/1
  Speed of Sound/1 -> a/1
  Position/1 -> Demux/1
  Demux/1 -> Terminator/1
  Demux/2 -> Terminator1/1
  Demux/3 -> OATemp/1, Density/1, Hp/1

== system SkywaveAutopilot/FlightGear/Lat,Lon,Elev Convertor ==
  Inp : Inport
  Demux : Demux  Outputs=3
      settings: DisplayOption=none
  Earth's radius : Constant  Value=6378137
  Gain : Gain
  Product : Product  Inputs=/*  SaturateOnIntegerOverflow=on  OutDataTypeStr=Inherit: Same as first input
  Product1 : Product  Inputs=*//  SaturateOnIntegerOverflow=on  OutDataTypeStr=Inherit: Same as first input
  Reference Altitude : Constant  Value=h_ref
  Reference Latitude : Constant  Value=lat_ref
  Reference Longitude : Constant  Value=long_ref
  Sum : Sum  Inputs=|++  SaturateOnIntegerOverflow=on
  Sum1 : Sum  Inputs=|++  SaturateOnIntegerOverflow=on
  Sum2 : Sum  Inputs=++|  SaturateOnIntegerOverflow=on
  Trigonometric Function : Trigonometry  Operator=cos
  Lon : Outport
  Lat : Outport  Port=2
  Ele : Outport  Port=3
  wires:
  Inp/1 -> Demux/1
  Sum/1 -> Ele/1
  Reference Altitude/1 -> Sum/2
  Earth's radius/1 -> Product/1, Product1/2
  Demux/1 -> Product/2
  Product/1 -> Sum2/2
  Sum2/1 -> Lat/1, Trigonometric Function/1
  Demux/3 -> Gain/1
  Demux/2 -> Product1/1
  Trigonometric Function/1 -> Product1/3
  Product1/1 -> Sum1/1
  Reference Longitude/1 -> Sum1/2
  Sum1/1 -> Lon/1
  Reference Latitude/1 -> Sum2/1
  Gain/1 -> Sum/1

== system SkywaveAutopilot/Longitudinal Autopilot/Climb ==
  RoC : Inport
  Action Port : ActionPort  ActionPortLabel=elseif(u1 < -100)
  Desired ROC : Constant  Value=1200
  Gain : Gain  Gain=1/60
  PID Controller1 : slpidlib/PID Controller  Controller=PID  Form=Parallel  TimeDomain=Continuous-time  UseExternalTs=off  SampleTime=-1  IntegratorMethod=Forward Euler  FilterMethod=Forward Euler  ControllerParametersSource=internal  P=-0.0746931727092318  I=-0.0439756497648282  UseKiTs=off  D=-0.0253317996869122  UseExternalDerivativeSource=off  N=12.6085681989155  UseFilter=on  TunerSelectOption=Transfer Function Based (PID Tuner App)  InitialConditionSource=internal  InitialConditionForIntegrator=0  InitialConditionForFilter=0  DifferentiatorICPrevScaledInput=0  ExternalReset=none  TrackingMode=off  Kt=1  LimitOutput=off  SatLimitsSource=internal  UpperSaturationLimit=inf  LowerSaturationLimit=-inf  LinearizeAsGain=on  AntiWindupMode=none  Kb=1  LimitIntegrator=off  UpperIntegratorSaturationLimit=inf  LowerIntegratorSaturationLimit=-inf  POutMin=[]  POutMax=[]  IOutMin=[]  IOutMax=[]  DOutMin=[]  DOutMax=[]  NOutMin=[]  NOutMax=[]  SumOutMin=[]  SumOutMax=[]  SaturationOutMin=[]  SaturationOutMax=[]  PParamMin=[]  PParamMax=[]  IParamMin=[]  IParamMax=[]  DParamMin=[]  DParamMax=[]  NParamMin=[]  NParamMax=[]  KbParamMin=[]  KbParamMax=[]  KtParamMin=[]  KtParamMax=[]  KbOutMin=[]  KbOutMax=[]  KtOutMin=[]  KtOutMax=[]  IntegratorOutMin=[]  IntegratorOutMax=[]  FilterOutMin=[]  FilterOutMax=[]  SumI1OutMin=[]  SumI1OutMax=[]  SumI2OutMin=[]  SumI2OutMax=[]  SumI3OutMin=[]  SumI3OutMax=[]  SumI4OutMin=[]  SumI4OutMax=[]  SumDOutMin=[]  SumDOutMax=[]  DifferentiatorOutMin=[]  DifferentiatorOutMax=[]  FilterDiffOutCoefMin=[]  FilterDiffOutCoefMax=[]  ReciprocalOutMin=[]  ReciprocalOutMax=[]  SumDenOutMin=[]  SumDenOutMax=[]  SumNumOutMin=[]  SumNumOutMax=[]  DivideOutMin=[]  DivideOutMax=[]  UdiffTsProdOutMin=[]  UdiffTsProdOutMax=[]  NTsProdOutMin=[]  NTsProdOutMax=[]  UintegralTsProdOutMin=[]  UintegralTsProdOutMax=[]  UngainTsProdOutMin=[]  UngainTsProdOutMax=[]  ClampingZeroOutDataTypeStr=Inherit: Inherit via back propagation  ClampingZeroOutMin=[]  ClampingZeroOutMax=[]  FilterDenConstantOutDataTypeStr=Inherit: Inherit via back propagation  FilterDenConstantOutMin=[]  FilterDenConstantOutMax=[]  PCopyOutDataTypeStr=Inherit: Inherit via back propagation  PCopyOutMin=[]  PCopyOutMax=[]  NCopyOutDataTypeStr=Inherit: Inherit via back propagation  NCopyOutMin=[]  NCopyOutMax=[]  IntegratorContinuousStateAttributes=''  IntegratorStateMustResolveToSignalObject=off  IntegratorRTWStateStorageClass=Auto  FilterContinuousStateAttributes=''  FilterStateMustResolveToSignalObject=off  FilterRTWStateStorageClass=Auto  ParallelPVariant=InternalParameters  IdealPVariant=Disabled  IVariant=InternalParameters  DVariant=InternalParameters  IntegratorVariant=Continuous  SatVariant=Disabled  AWVariant=Passthrough  PCopyVariant=Disabled  TRVariant=Disabled  FdbkBlocksVariant=Forward  IdealPFdbkVariant=Disabled  SatFdbkVariant=Disabled  DerivativeFilterVariant=ContFilter  NVariant=InternalParameters  NCopyVariant=Disabled  FilterICVariant=InternalICsFilter  IntegratorICVariant=InternalICs  ExternalResetVariant=Disabled  TRSumVariant=Passthrough  SumFdbkVariant=Disabled  SumVariant=Sum_PID  TsampFilterVariant=InternalTs  TsampNgainVariant=Passthrough  TsampIntegralVariant=Disabled_SignalSpec  ExternalSaturationOutDataTypeStr=Inherit: Same as second input  DerivativeSourceVariant=ErrorSignal  PreIntVariant=InternalPreInt
  PID ControllerGood : slpidlib/PID Controller  Controller=PID  Form=Parallel  TimeDomain=Continuous-time  UseExternalTs=off  SampleTime=-1  IntegratorMethod=Forward Euler  FilterMethod=Forward Euler  ControllerParametersSource=internal  P=-0.000923867755210005  I=-0.000116592048001939  UseKiTs=off  D=0  UseExternalDerivativeSource=off  N=100  UseFilter=on  TunerSelectOption=Transfer Function Based (PID Tuner App)  InitialConditionSource=internal  InitialConditionForIntegrator=0  InitialConditionForFilter=0  DifferentiatorICPrevScaledInput=0  ExternalReset=none  TrackingMode=off  Kt=1  LimitOutput=off  SatLimitsSource=internal  UpperSaturationLimit=inf  LowerSaturationLimit=-inf  LinearizeAsGain=on  AntiWindupMode=none  Kb=1  LimitIntegrator=off  UpperIntegratorSaturationLimit=inf  LowerIntegratorSaturationLimit=-inf  POutMin=[]  POutMax=[]  IOutMin=[]  IOutMax=[]  DOutMin=[]  DOutMax=[]  NOutMin=[]  NOutMax=[]  SumOutMin=[]  SumOutMax=[]  SaturationOutMin=[]  SaturationOutMax=[]  PParamMin=[]  PParamMax=[]  IParamMin=[]  IParamMax=[]  DParamMin=[]  DParamMax=[]  NParamMin=[]  NParamMax=[]  KbParamMin=[]  KbParamMax=[]  KtParamMin=[]  KtParamMax=[]  KbOutMin=[]  KbOutMax=[]  KtOutMin=[]  KtOutMax=[]  IntegratorOutMin=[]  IntegratorOutMax=[]  FilterOutMin=[]  FilterOutMax=[]  SumI1OutMin=[]  SumI1OutMax=[]  SumI2OutMin=[]  SumI2OutMax=[]  SumI3OutMin=[]  SumI3OutMax=[]  SumI4OutMin=[]  SumI4OutMax=[]  SumDOutMin=[]  SumDOutMax=[]  DifferentiatorOutMin=[]  DifferentiatorOutMax=[]  FilterDiffOutCoefMin=[]  FilterDiffOutCoefMax=[]  ReciprocalOutMin=[]  ReciprocalOutMax=[]  SumDenOutMin=[]  SumDenOutMax=[]  SumNumOutMin=[]  SumNumOutMax=[]  DivideOutMin=[]  DivideOutMax=[]  UdiffTsProdOutMin=[]  UdiffTsProdOutMax=[]  NTsProdOutMin=[]  NTsProdOutMax=[]  UintegralTsProdOutMin=[]  UintegralTsProdOutMax=[]  UngainTsProdOutMin=[]  UngainTsProdOutMax=[]  ClampingZeroOutDataTypeStr=Inherit: Inherit via back propagation  ClampingZeroOutMin=[]  ClampingZeroOutMax=[]  FilterDenConstantOutDataTypeStr=Inherit: Inherit via back propagation  FilterDenConstantOutMin=[]  FilterDenConstantOutMax=[]  PCopyOutDataTypeStr=Inherit: Inherit via back propagation  PCopyOutMin=[]  PCopyOutMax=[]  NCopyOutDataTypeStr=Inherit: Inherit via back propagation  NCopyOutMin=[]  NCopyOutMax=[]  IntegratorContinuousStateAttributes=''  IntegratorStateMustResolveToSignalObject=off  IntegratorRTWStateStorageClass=Auto  FilterContinuousStateAttributes=''  FilterStateMustResolveToSignalObject=off  FilterRTWStateStorageClass=Auto  ParallelPVariant=InternalParameters  IdealPVariant=Disabled  IVariant=InternalParameters  DVariant=InternalParameters  IntegratorVariant=Continuous  SatVariant=Disabled  AWVariant=Passthrough  PCopyVariant=Disabled  TRVariant=Disabled  FdbkBlocksVariant=Forward  IdealPFdbkVariant=Disabled  SatFdbkVariant=Disabled  DerivativeFilterVariant=ContFilter  NVariant=InternalParameters  NCopyVariant=Disabled  FilterICVariant=InternalICsFilter  IntegratorICVariant=InternalICs  ExternalResetVariant=Disabled  TRSumVariant=Passthrough  SumFdbkVariant=Disabled  SumVariant=Sum_PID  TsampFilterVariant=InternalTs  TsampNgainVariant=Passthrough  TsampIntegralVariant=Disabled_SignalSpec  ExternalSaturationOutDataTypeStr=Inherit: Same as second input  DerivativeSourceVariant=ErrorSignal  PreIntVariant=InternalPreInt
  Signal : Constant  Value=3
  Sum : Sum  Inputs=|+-
  Out1 : Outport
  Debug : Outport  Port=2
  wires:
  Desired ROC/1 -> Gain/1
  Signal/1 -> Debug/1
  RoC/1 -> Sum/1
  Gain/1 -> Sum/2
  Sum/1 -> PID Controller1/1
  PID Controller1/1 -> Out1/1

== system SkywaveAutopilot/Longitudinal Autopilot/Descend ==
  RoC : Inport
  Action Port : ActionPort  ActionPortLabel=if(u1 > 100)
  Desired ROC : Constant  Value=-1200
  Gain : Gain  Gain=1/60
  PID Controller1 : slpidlib/PID Controller  Controller=PID  Form=Parallel  TimeDomain=Continuous-time  UseExternalTs=off  SampleTime=-1  IntegratorMethod=Forward Euler  FilterMethod=Forward Euler  ControllerParametersSource=internal  P=-0.0746931727092318  I=-0.0439756497648282  UseKiTs=off  D=-0.0253317996869122  UseExternalDerivativeSource=off  N=12.6085681989155  UseFilter=on  TunerSelectOption=Transfer Function Based (PID Tuner App)  InitialConditionSource=internal  InitialConditionForIntegrator=0  InitialConditionForFilter=0  DifferentiatorICPrevScaledInput=0  ExternalReset=none  TrackingMode=off  Kt=1  LimitOutput=off  SatLimitsSource=internal  UpperSaturationLimit=inf  LowerSaturationLimit=-inf  LinearizeAsGain=on  AntiWindupMode=none  Kb=1  LimitIntegrator=off  UpperIntegratorSaturationLimit=inf  LowerIntegratorSaturationLimit=-inf  POutMin=[]  POutMax=[]  IOutMin=[]  IOutMax=[]  DOutMin=[]  DOutMax=[]  NOutMin=[]  NOutMax=[]  SumOutMin=[]  SumOutMax=[]  SaturationOutMin=[]  SaturationOutMax=[]  PParamMin=[]  PParamMax=[]  IParamMin=[]  IParamMax=[]  DParamMin=[]  DParamMax=[]  NParamMin=[]  NParamMax=[]  KbParamMin=[]  KbParamMax=[]  KtParamMin=[]  KtParamMax=[]  KbOutMin=[]  KbOutMax=[]  KtOutMin=[]  KtOutMax=[]  IntegratorOutMin=[]  IntegratorOutMax=[]  FilterOutMin=[]  FilterOutMax=[]  SumI1OutMin=[]  SumI1OutMax=[]  SumI2OutMin=[]  SumI2OutMax=[]  SumI3OutMin=[]  SumI3OutMax=[]  SumI4OutMin=[]  SumI4OutMax=[]  SumDOutMin=[]  SumDOutMax=[]  DifferentiatorOutMin=[]  DifferentiatorOutMax=[]  FilterDiffOutCoefMin=[]  FilterDiffOutCoefMax=[]  ReciprocalOutMin=[]  ReciprocalOutMax=[]  SumDenOutMin=[]  SumDenOutMax=[]  SumNumOutMin=[]  SumNumOutMax=[]  DivideOutMin=[]  DivideOutMax=[]  UdiffTsProdOutMin=[]  UdiffTsProdOutMax=[]  NTsProdOutMin=[]  NTsProdOutMax=[]  UintegralTsProdOutMin=[]  UintegralTsProdOutMax=[]  UngainTsProdOutMin=[]  UngainTsProdOutMax=[]  ClampingZeroOutDataTypeStr=Inherit: Inherit via back propagation  ClampingZeroOutMin=[]  ClampingZeroOutMax=[]  FilterDenConstantOutDataTypeStr=Inherit: Inherit via back propagation  FilterDenConstantOutMin=[]  FilterDenConstantOutMax=[]  PCopyOutDataTypeStr=Inherit: Inherit via back propagation  PCopyOutMin=[]  PCopyOutMax=[]  NCopyOutDataTypeStr=Inherit: Inherit via back propagation  NCopyOutMin=[]  NCopyOutMax=[]  IntegratorContinuousStateAttributes=''  IntegratorStateMustResolveToSignalObject=off  IntegratorRTWStateStorageClass=Auto  FilterContinuousStateAttributes=''  FilterStateMustResolveToSignalObject=off  FilterRTWStateStorageClass=Auto  ParallelPVariant=InternalParameters  IdealPVariant=Disabled  IVariant=InternalParameters  DVariant=InternalParameters  IntegratorVariant=Continuous  SatVariant=Disabled  AWVariant=Passthrough  PCopyVariant=Disabled  TRVariant=Disabled  FdbkBlocksVariant=Forward  IdealPFdbkVariant=Disabled  SatFdbkVariant=Disabled  DerivativeFilterVariant=ContFilter  NVariant=InternalParameters  NCopyVariant=Disabled  FilterICVariant=InternalICsFilter  IntegratorICVariant=InternalICs  ExternalResetVariant=Disabled  TRSumVariant=Passthrough  SumFdbkVariant=Disabled  SumVariant=Sum_PID  TsampFilterVariant=InternalTs  TsampNgainVariant=Passthrough  TsampIntegralVariant=Disabled_SignalSpec  ExternalSaturationOutDataTypeStr=Inherit: Same as second input  DerivativeSourceVariant=ErrorSignal  PreIntVariant=InternalPreInt
  PID ControllerGood : slpidlib/PID Controller  Controller=PID  Form=Parallel  TimeDomain=Continuous-time  UseExternalTs=off  SampleTime=-1  IntegratorMethod=Forward Euler  FilterMethod=Forward Euler  ControllerParametersSource=internal  P=-0.000923867755210005  I=-0.000116592048001939  UseKiTs=off  D=0  UseExternalDerivativeSource=off  N=100  UseFilter=on  TunerSelectOption=Transfer Function Based (PID Tuner App)  InitialConditionSource=internal  InitialConditionForIntegrator=0  InitialConditionForFilter=0  DifferentiatorICPrevScaledInput=0  ExternalReset=none  TrackingMode=off  Kt=1  LimitOutput=off  SatLimitsSource=internal  UpperSaturationLimit=inf  LowerSaturationLimit=-inf  LinearizeAsGain=on  AntiWindupMode=none  Kb=1  LimitIntegrator=off  UpperIntegratorSaturationLimit=inf  LowerIntegratorSaturationLimit=-inf  POutMin=[]  POutMax=[]  IOutMin=[]  IOutMax=[]  DOutMin=[]  DOutMax=[]  NOutMin=[]  NOutMax=[]  SumOutMin=[]  SumOutMax=[]  SaturationOutMin=[]  SaturationOutMax=[]  PParamMin=[]  PParamMax=[]  IParamMin=[]  IParamMax=[]  DParamMin=[]  DParamMax=[]  NParamMin=[]  NParamMax=[]  KbParamMin=[]  KbParamMax=[]  KtParamMin=[]  KtParamMax=[]  KbOutMin=[]  KbOutMax=[]  KtOutMin=[]  KtOutMax=[]  IntegratorOutMin=[]  IntegratorOutMax=[]  FilterOutMin=[]  FilterOutMax=[]  SumI1OutMin=[]  SumI1OutMax=[]  SumI2OutMin=[]  SumI2OutMax=[]  SumI3OutMin=[]  SumI3OutMax=[]  SumI4OutMin=[]  SumI4OutMax=[]  SumDOutMin=[]  SumDOutMax=[]  DifferentiatorOutMin=[]  DifferentiatorOutMax=[]  FilterDiffOutCoefMin=[]  FilterDiffOutCoefMax=[]  ReciprocalOutMin=[]  ReciprocalOutMax=[]  SumDenOutMin=[]  SumDenOutMax=[]  SumNumOutMin=[]  SumNumOutMax=[]  DivideOutMin=[]  DivideOutMax=[]  UdiffTsProdOutMin=[]  UdiffTsProdOutMax=[]  NTsProdOutMin=[]  NTsProdOutMax=[]  UintegralTsProdOutMin=[]  UintegralTsProdOutMax=[]  UngainTsProdOutMin=[]  UngainTsProdOutMax=[]  ClampingZeroOutDataTypeStr=Inherit: Inherit via back propagation  ClampingZeroOutMin=[]  ClampingZeroOutMax=[]  FilterDenConstantOutDataTypeStr=Inherit: Inherit via back propagation  FilterDenConstantOutMin=[]  FilterDenConstantOutMax=[]  PCopyOutDataTypeStr=Inherit: Inherit via back propagation  PCopyOutMin=[]  PCopyOutMax=[]  NCopyOutDataTypeStr=Inherit: Inherit via back propagation  NCopyOutMin=[]  NCopyOutMax=[]  IntegratorContinuousStateAttributes=''  IntegratorStateMustResolveToSignalObject=off  IntegratorRTWStateStorageClass=Auto  FilterContinuousStateAttributes=''  FilterStateMustResolveToSignalObject=off  FilterRTWStateStorageClass=Auto  ParallelPVariant=InternalParameters  IdealPVariant=Disabled  IVariant=InternalParameters  DVariant=InternalParameters  IntegratorVariant=Continuous  SatVariant=Disabled  AWVariant=Passthrough  PCopyVariant=Disabled  TRVariant=Disabled  FdbkBlocksVariant=Forward  IdealPFdbkVariant=Disabled  SatFdbkVariant=Disabled  DerivativeFilterVariant=ContFilter  NVariant=InternalParameters  NCopyVariant=Disabled  FilterICVariant=InternalICsFilter  IntegratorICVariant=InternalICs  ExternalResetVariant=Disabled  TRSumVariant=Passthrough  SumFdbkVariant=Disabled  SumVariant=Sum_PID  TsampFilterVariant=InternalTs  TsampNgainVariant=Passthrough  TsampIntegralVariant=Disabled_SignalSpec  ExternalSaturationOutDataTypeStr=Inherit: Same as second input  DerivativeSourceVariant=ErrorSignal  PreIntVariant=InternalPreInt
  Signal : Constant
  Sum : Sum  Inputs=|+-
  del_e : Outport
  Debug : Outport  Port=2
  wires:
  RoC/1 -> Sum/1
  Desired ROC/1 -> Gain/1
  Signal/1 -> Debug/1
  Gain/1 -> Sum/2
  Sum/1 -> PID Controller1/1
  PID Controller1/1 -> del_e/1
